simulink model "fm_ddc_diff"  (Simulink 7.7)
settings: Solver=FixedStepDiscrete  SolverMode=SingleTasking  StartTime=0.0  StopTime=2e5/SR  RelTol=1e-3
model workspace (MAT data in the model file):
  synDspToolFileName = 'c:\demo\ddc31\gsm_ddc.mdl'
  synDspToolHandle : num (value not decoded)
PreLoadFcn:
  | SR=80e6 ;%Sample rate variable
  | IF=103.9e6
  | % Create filters normalized to sample rate
  | cfir_passband_edge = 105e3/(SR/128)*2;
  | %mfir_pass_edge = 80e3/(SR/128)*2;
  | %mfir_stopb_strt = 100e3/(SR/128)*2;
  | mfir_pass_edge  = 100e3/(SR/128)*2;
  | mfir_stopb_strt = 130e3/(SR/128)*2;
  | 
  | %Create input stimulus and plot so we can see
  | %All are centered around a 7mhz carrier
  | %Two sin in middle and edge of passband
  | ddc_in = .8*sin(2*pi*(40e3+IF)/SR*(1:20e4)) + .6*sin(2*pi*(80e3+IF)/SR*(1:20e4));
  | %sin in adjacent channel
  | ddc_in = ddc_in + .9*sin(2*pi*(100e3+IF)/SR*(1:20e4)) + 1.2*sin(2*pi*(120e3+IF)/SR*(1:20e4))+ 3.9*sin(2*pi*(130e3+IF)/SR*(1:20e4));
  | %sin in distant channels
  | ddc_in = ddc_in + 1.1*sin(2*pi*(487e3+IF)/SR*(1:20e4)) + 2.1*sin(2*pi*(22e6+IF)/SR*(1:20e4)) ;
  | randn('state',171);
  | ddc_in = awgn(ddc_in,10,0);     %add some noise
  | fft_size=2^16;
  | fddc_in = fft(ddc_in(1:fft_size-1));  %need high resolution fft to resolve peaks
  | %sp_view_L=ceil(2*IF/SR*fft_size);
  | %sp_view_H=ceil(2*(IF+1e6)/SR*fft_size);
  | %plot(20*log(abs(fddc_in(sp_view_L:sp_view_H)/max(abs(fddc_in)))))%plot just the section we want to see
  | %grid;
undefined symbols (not defined in the file or in its folder): One, sided, syn_get_coefs
libraries: shlslibv1 x27, dspsnks4 x4, dspsrcs4 x1
settings Model: MinMaxOverflowLogging=OverflowOnly  synDspstartup=OK  Creator=dirk  LastModifiedBy=Administrator
settings DataIOCC: SaveOutput=off  SignalLogging=off  SaveTime=off
settings OptimizationCC: InlineParams=on  InitFltsAndDblsToZero=on
settings DebuggingCC: AlgebraicLoopMsg=error  SaveWithParameterizedLinksMsg=none  SignalResolutionControl=TryResolveAllWithWarning  InheritedTsInSrcMsg=none  MultiTaskDSMMsg=warning  MultiTaskCondExecSysMsg=none  StrictBusMsg=Warning
settings RTWCC: IncludeERTFirstTime=on
settings GRTTargetCC: TargetFcnLib=ansi_tfl_tmw.mat

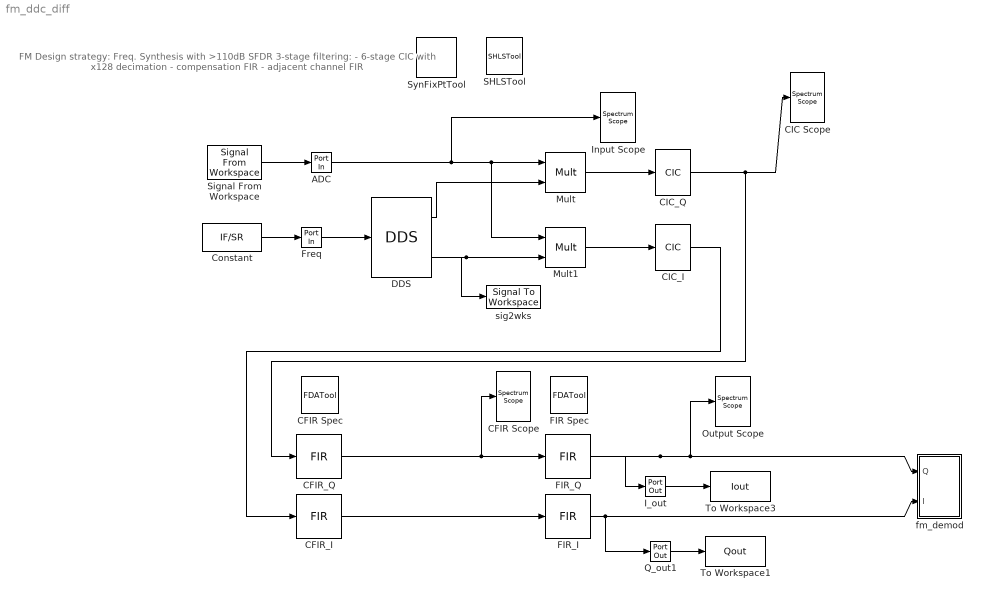
== system fm_ddc_diff ==
  note: FM Design strategy:
      | Freq.  Synthesis with >110dB SFDR
      | 3-stage filtering:
      | - 6-stage CIC with x128 decimation
      | -  compensation FIR
      | -  adjacent channel FIR
  ADC : shlslibv1/Ports & Subsystems/Port In  syn_out_wl=14  syn_out_fl=12  syn_out_dt=signed  syn_out_st=1/SR  syn_capture=on  syn_register=on  syn_out_sat=off  syn_out_rnd=on  synBlockType=port  synLatency=1  synBlockId=0
  CFIR Scope : dspsnks4/Spectrum Scope  SystemSampleTime=-1  ScopeProperties=on  Domain=Frequency  HorizSpan=1  UseBuffer=on  BufferSize=2^9  Overlap=2^8  TreatMby1Signals=M channels  inpFftLenInherit=off  FFTlength=128  numAvg=17  DisplayProperties=off  AxisGrid=on  Memory=off  FrameNumber=on  AxisLegend=off  AxisZoom=off  OpenScopeAtSimStart=on  OpenScopeImmediately=off  FigPos=[785 600 380 380]  AxisProperties=off  XUnits=Hertz  XRange=One-sided ([0...Fs/2])  XDisplay=0  InheritXIncr=off  XIncr=128/SR  XLabel=Samples  XLimit=Auto  YUnits=dBW/Hertz  XMax=1  XMin=0  YLabel=Magnitude-squared, dB  LineProperties=off  wintypeSpecScope=Hann  RsSpecScope=50  betaSpecScope=5  winsampSpecScope=Periodic  XAxisParamsVer=6.8  isFrameUpgraded=on
      settings: YMin=-93.2061394535487  YMax=-7.27904806219149
  CFIR Spec : shlslibv1/Filtering/FDATool  SystemSampleTime=-1  synBlockType=tool
  CFIR_I : shlslibv1/Filtering/FIR  syn_coef_vec=syn_get_coefs('CFIR Spec')  syn_coef_fl=8  syn_coef_rnd=Nearest  syn_show_q=off  syn_dp_f=Automatic  syn_dp_wl=16  syn_dp_fl=8  syn_dp_sat=off  syn_dp_rnd=Floor (Truncate)  syn_out_f=Specify  syn_out_wl=16  syn_out_fl=13  syn_out_dt=signed  syn_out_sat=off  syn_out_rnd=Floor (Truncate)  syn_rst_port=off  syn_en_port=off  synBlockType=primitive  synLatency=0  synBlockId=80
  CFIR_Q : shlslibv1/Filtering/FIR  syn_coef_vec=syn_get_coefs('CFIR Spec')  syn_coef_fl=8  syn_coef_rnd=Nearest  syn_show_q=off  syn_dp_f=Automatic  syn_dp_wl=16  syn_dp_fl=8  syn_dp_sat=off  syn_dp_rnd=Floor (Truncate)  syn_out_f=Specify  syn_out_wl=16  syn_out_fl=13  syn_out_dt=signed  syn_out_sat=off  syn_out_rnd=Floor (Truncate)  syn_rst_port=off  syn_en_port=off  synBlockType=primitive  synLatency=0  synBlockId=80
  CIC Scope : dspsnks4/Spectrum Scope  SystemSampleTime=-1  ScopeProperties=on  Domain=Frequency  HorizSpan=1  UseBuffer=on  BufferSize=2^10  Overlap=2^9  TreatMby1Signals=M channels  inpFftLenInherit=off  FFTlength=128  numAvg=16  DisplayProperties=off  AxisGrid=on  Memory=off  FrameNumber=on  AxisLegend=off  AxisZoom=off  OpenScopeAtSimStart=on  OpenScopeImmediately=off  FigPos=[395 600 380 380]  AxisProperties=off  XUnits=Hertz  XRange=One-sided ([0...Fs/2])  XDisplay=0  InheritXIncr=off  XIncr=128/SR  XLabel=Samples  XLimit=Auto  YUnits=dBW/Hertz  XMax=1  XMin=0  YLabel=Magnitude-squared, dB  LineProperties=off  wintypeSpecScope=Hann  RsSpecScope=50  betaSpecScope=5  winsampSpecScope=Periodic  XAxisParamsVer=6.8  isFrameUpgraded=on
      settings: YMin=-66.8830492621563  YMax=-9.39744350931665
  CIC_I : shlslibv1/Filtering/CIC  SystemSampleTime=-1  syn_cic_type=Decimator  syn_m_val=1  syn_r_val=128  syn_n_val=6  syn_out_f=Specify  syn_out_wl=18  syn_out_fl=16  syn_out_dt=signed  syn_out_sat=off  syn_out_rnd=off  syn_rst_port=off  syn_en_port=off  synBlockType=custom  synLatency=1
      settings: AttributesFormatString=1.0000000000
  CIC_Q : shlslibv1/Filtering/CIC  SystemSampleTime=-1  syn_cic_type=Decimator  syn_m_val=1  syn_r_val=128  syn_n_val=6  syn_out_f=Specify  syn_out_wl=18  syn_out_fl=16  syn_out_dt=signed  syn_out_sat=off  syn_out_rnd=off  syn_rst_port=off  syn_en_port=off  synBlockType=custom  synLatency=1
      settings: AttributesFormatString=1.0000000000
  Constant : Constant  Value=IF/SR  SampleTime=1/SR
  DDS : shlslibv1/Sources/DDS  SystemSampleTime=-1  syn_dds_opr=sin&cos  syn_dds_meth=CORDIC  syn_freq_port=port  syn_freq_val=5/24  syn_fm_port=none  syn_fm_val=0  syn_pm_port=none  syn_pm_val=0  syn_pdither_opr=on  syn_pdither_bits=3  syn_rst_port=off  syn_en_port=off  syn_freq_prec=2^-32  syn_phase_prec=2^-18  syn_dds_wl=18  syn_dds_st=3/208e6  synBlockType=custom  synLatency=20
  FIR Spec : shlslibv1/Filtering/FDATool  SystemSampleTime=-1  synBlockType=tool
  FIR_I : shlslibv1/Filtering/FIR  syn_coef_vec=syn_get_coefs('FIR Spec')  syn_coef_fl=8  syn_coef_rnd=Nearest  syn_show_q=off  syn_dp_f=Automatic  syn_dp_wl=16  syn_dp_fl=8  syn_dp_sat=off  syn_dp_rnd=Floor (Truncate)  syn_out_f=Specify  syn_out_wl=16  syn_out_fl=12  syn_out_dt=signed  syn_out_sat=off  syn_out_rnd=Floor (Truncate)  syn_rst_port=off  syn_en_port=off  synBlockType=primitive  synLatency=0  synBlockId=80
  FIR_Q : shlslibv1/Filtering/FIR  syn_coef_vec=syn_get_coefs('FIR Spec')  syn_coef_fl=8  syn_coef_rnd=Nearest  syn_show_q=off  syn_dp_f=Automatic  syn_dp_wl=16  syn_dp_fl=8  syn_dp_sat=off  syn_dp_rnd=Floor (Truncate)  syn_out_f=Specify  syn_out_wl=16  syn_out_fl=12  syn_out_dt=signed  syn_out_sat=off  syn_out_rnd=Floor (Truncate)  syn_rst_port=off  syn_en_port=off  synBlockType=primitive  synLatency=0  synBlockId=80
  Freq : shlslibv1/Ports & Subsystems/Port In  syn_out_wl=32  syn_out_fl=32  syn_out_dt=unsigned  syn_out_st=1/SR  syn_capture=on  syn_register=on  syn_out_sat=off  syn_out_rnd=on  synBlockType=port  synLatency=1  synBlockId=0
  I_out : shlslibv1/Ports & Subsystems/Port Out  syn_capture=on  syn_register=on  synBlockType=port  synLatency=1  synBlockId=1
  Input Scope : dspsnks4/Spectrum Scope  SystemSampleTime=-1  ScopeProperties=on  Domain=Frequency  HorizSpan=1  UseBuffer=on  BufferSize=2^12  Overlap=2^11  TreatMby1Signals=M channels  inpFftLenInherit=off  FFTlength=128  numAvg=16  DisplayProperties=off  AxisGrid=on  Memory=off  FrameNumber=on  AxisLegend=off  AxisZoom=off  OpenScopeAtSimStart=on  OpenScopeImmediately=off  FigPos=[5 600 380 380]  AxisProperties=off  XUnits=Hertz  XRange=One-sided ([0...Fs/2])  XDisplay=0  InheritXIncr=off  XIncr=1/SR  XLabel=Samples  XLimit=Auto  YUnits=dBW/Hertz  XMax=1  XMin=0  YLabel=Magnitude-squared, dB  LineProperties=off  wintypeSpecScope=Hann  RsSpecScope=50  betaSpecScope=5  winsampSpecScope=Periodic  XAxisParamsVer=6.8  isFrameUpgraded=on
      settings: YMin=-19.5299787439029  YMax=9.72164383894065
  Mult : shlslibv1/Math Functions/Mult  syn_out_f=Specify  syn_out_wl=18  syn_out_fl=16  syn_out_dt=signed  syn_out_sat=off  syn_out_rnd=Floor (Truncate)  syn_inh_port=off  syn_inh_st=off  syn_inh_stf=1  synBlockType=primitive  synLatency=0  synBlockId=3  syn_opr_mode=1
  Mult1 : shlslibv1/Math Functions/Mult  syn_out_f=Specify  syn_out_wl=18  syn_out_fl=16  syn_out_dt=signed  syn_out_sat=off  syn_out_rnd=Floor (Truncate)  syn_inh_port=off  syn_inh_st=off  syn_inh_stf=1  synBlockType=primitive  synLatency=0  synBlockId=3  syn_opr_mode=1
  Output Scope : dspsnks4/Spectrum Scope  SystemSampleTime=-1  ScopeProperties=on  Domain=Frequency  HorizSpan=1  UseBuffer=on  BufferSize=2^8  Overlap=2^7  TreatMby1Signals=M channels  inpFftLenInherit=off  FFTlength=128  numAvg=10  DisplayProperties=off  AxisGrid=on  Memory=off  FrameNumber=on  AxisLegend=off  AxisZoom=off  OpenScopeAtSimStart=on  OpenScopeImmediately=off  FigPos=[785 200 380 380]  AxisProperties=off  XUnits=Hertz  XRange=One-sided ([0...Fs/2])  XDisplay=0  InheritXIncr=off  XIncr=128/SR  XLabel=Samples  XLimit=Auto  YUnits=dBW/Hertz  XMax=1  XMin=0  YLabel=Magnitude-squared, dB  LineProperties=off  wintypeSpecScope=Hann  RsSpecScope=50  betaSpecScope=5  winsampSpecScope=Periodic  XAxisParamsVer=6.8  isFrameUpgraded=on
      settings: YMin=-93.2061394535487  YMax=-7.27904806219149
  Q_out1 : shlslibv1/Ports & Subsystems/Port Out  syn_capture=on  syn_register=on  synBlockType=port  synLatency=1  synBlockId=1
  SHLSTool : shlslibv1/SHLSTool  SystemSampleTime=-1  synBlockType=tool  syn_dsp_mode=FPGA
  Signal From Workspace : dspsrcs4/Signal From Workspace  SystemSampleTime=-1  X=ddc_in  Ts=1/SR  nsamps=1  OutputAfterFinalValue=Cyclic repetition  ignoreOrWarnInputAndFrameLengths=off
  SynFixPtTool : shlslibv1/SynFixPtTool  SystemSampleTime=-1  synBlockType=tool
  To Workspace1 : ToWorkspace  VariableName=Qout  SampleTime=-1  SaveFormat=Structure With Time
  To Workspace3 : ToWorkspace  VariableName=Iout  SampleTime=-1  SaveFormat=Structure With Time
  fm_demod : Subsystem
  sig2wks : SignalToWorkspace  VariableName=dds_out  SaveFormat=Array
      settings: CopyFcn=dspblkcopystw(gcbh);
  wires:
  ADC/1 -> Mult/1, Mult1/1, Input Scope/1
  Constant/1 -> Freq/1
  Freq/1 -> DDS/1
  DDS/1 -> Mult/2
  DDS/2 -> Mult1/2, sig2wks/1
  CIC_Q/1 -> CFIR_Q/1, CIC Scope/1
  CFIR_Q/1 -> FIR_Q/1, CFIR Scope/1
  CFIR_I/1 -> FIR_I/1
  CIC_I/1 -> CFIR_I/1
  FIR_Q/1 -> Output Scope/1, fm_demod/1(Q), I_out/1
  FIR_I/1 -> Q_out1/1, fm_demod/2(I)
  Mult1/1 -> CIC_I/1
  Mult/1 -> CIC_Q/1
  Signal From Workspace/1 -> ADC/1
  I_out/1 -> To Workspace3/1
  Q_out1/1 -> To Workspace1/1

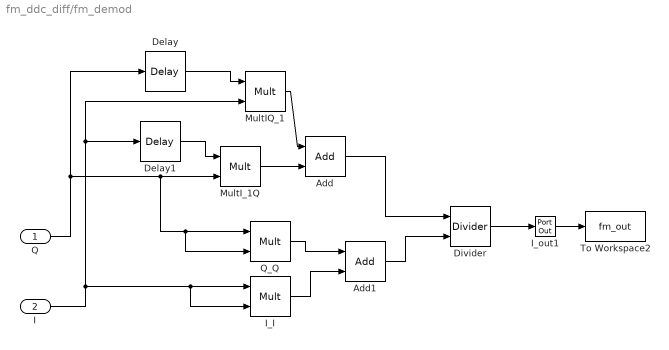
== system fm_ddc_diff/fm_demod ==
  Q : Inport
  I : Inport  Port=2
  Add : shlslibv1/Math Functions/Add  syn_add_opr=+-  syn_out_f=Full Precision  syn_out_wl=16  syn_out_fl=8  syn_out_dt=signed  syn_out_sat=off  syn_out_rnd=Floor (Truncate)  synBlockType=primitive  synLatency=0  synBlockId=96  syn_sum_of_rows=off  syn_inh_port=off  syn_inh_st=off  syn_inh_stf=1
  Add1 : shlslibv1/Math Functions/Add  syn_add_opr=++  syn_out_f=Full Precision  syn_out_wl=16  syn_out_fl=8  syn_out_dt=signed  syn_out_sat=off  syn_out_rnd=Floor (Truncate)  synBlockType=primitive  synLatency=0  synBlockId=96  syn_sum_of_rows=off  syn_inh_port=off  syn_inh_st=off  syn_inh_stf=1
  Delay : shlslibv1/Memories/Delay  syn_delay_val=1  synBlockType=primitive  synLatency=1  synBlockId=104
  Delay1 : shlslibv1/Memories/Delay  syn_delay_val=1  synBlockType=primitive  synLatency=1  synBlockId=104
  Divider : shlslibv1/Math Functions/Divider  syn_div_mode=Normal  syn_out_f=Specify  syn_out_wl=16  syn_out_fl=8  syn_out_dt=signed  syn_out_sat=off  syn_out_rnd=off  syn_out_dbz=off  synBlockType=primitive  synLatency=0  synBlockId=152
  I_I : shlslibv1/Math Functions/Mult  syn_out_f=Specify  syn_out_wl=18  syn_out_fl=16  syn_out_dt=signed  syn_out_sat=off  syn_out_rnd=Floor (Truncate)  syn_inh_port=off  syn_inh_st=off  syn_inh_stf=1  synBlockType=primitive  synLatency=0  synBlockId=3  syn_opr_mode=1
  I_out1 : shlslibv1/Ports & Subsystems/Port Out  syn_capture=on  syn_register=on  synBlockType=port  synLatency=1  synBlockId=1
  MultIQ_1 : shlslibv1/Math Functions/Mult  syn_out_f=Specify  syn_out_wl=18  syn_out_fl=16  syn_out_dt=signed  syn_out_sat=off  syn_out_rnd=Floor (Truncate)  syn_inh_port=off  syn_inh_st=off  syn_inh_stf=1  synBlockType=primitive  synLatency=0  synBlockId=3  syn_opr_mode=1
  MultI_1Q : shlslibv1/Math Functions/Mult  syn_out_f=Specify  syn_out_wl=18  syn_out_fl=16  syn_out_dt=signed  syn_out_sat=off  syn_out_rnd=Floor (Truncate)  syn_inh_port=off  syn_inh_st=off  syn_inh_stf=1  synBlockType=primitive  synLatency=0  synBlockId=3  syn_opr_mode=1
  Q_Q : shlslibv1/Math Functions/Mult  syn_out_f=Specify  syn_out_wl=18  syn_out_fl=16  syn_out_dt=signed  syn_out_sat=off  syn_out_rnd=Floor (Truncate)  syn_inh_port=off  syn_inh_st=off  syn_inh_stf=1  synBlockType=primitive  synLatency=0  synBlockId=3  syn_opr_mode=1
  To Workspace2 : ToWorkspace  VariableName=fm_out  SampleTime=-1  SaveFormat=Structure With Time
  wires:
  Divider/1 -> I_out1/1
  I_out1/1 -> To Workspace2/1
  Delay1/1 -> MultI_1Q/1
  Delay/1 -> MultIQ_1/1
  MultIQ_1/1 -> Add/1
  MultI_1Q/1 -> Add/2
  Q_Q/1 -> Add1/1
  I_I/1 -> Add1/2
  Add/1 -> Divider/1
  Add1/1 -> Divider/2
  Q/1 -> Delay/1, MultI_1Q/2, Q_Q/1, Q_Q/2
  I/1 -> MultIQ_1/2, Delay1/1, I_I/1, I_I/2
